simulink model "expr2_1"  (R2021b)
settings: Solver=VariableStepAuto  StartTime=0.0  StopTime=10.0  RelTol=1e-3
settings Model: Creator=86137  LastModifiedBy=86137

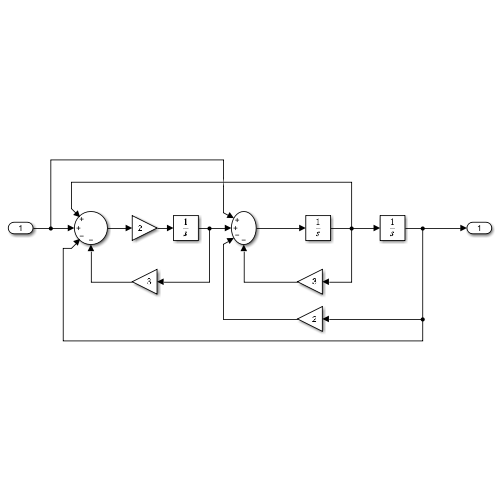
[thumbnail: Simulink's stored preview of the top-level diagram]
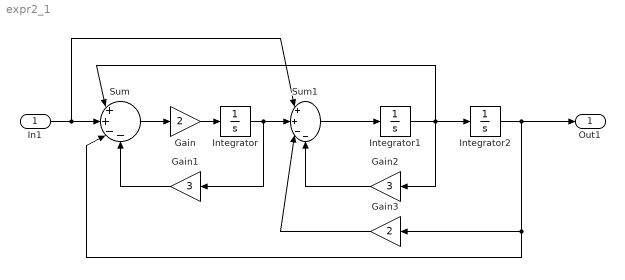
== system expr2_1 ==
  In1 : Inport
  Gain : Gain  Gain=2
  Gain1 : Gain  Gain=3
  Gain2 : Gain  Gain=3
  Gain3 : Gain  Gain=2
  Integrator : Integrator
  Integrator1 : Integrator
  Integrator2 : Integrator
  Sum : Sum  Inputs=|++--
  Sum1 : Sum  Inputs=|++--
  Out1 : Outport
  wires:
  In1/1 -> Sum1/1, Sum/2
  Integrator/1 -> Gain1/1, Sum1/2
  Sum/1 -> Gain/1
  Gain/1 -> Integrator/1
  Gain1/1 -> Sum/4
  Sum1/1 -> Integrator1/1
  Integrator1/1 -> Sum/1, Gain2/1, Integrator2/1
  Gain2/1 -> Sum1/4
  Integrator2/1 -> Gain3/1, Sum/3, Out1/1
  Gain3/1 -> Sum1/3
